simulink model "MIMO_MFDM_Mdl_Zenith"  (R2023b)
settings: Solver=FixedStepAuto  StartTime=0.0  StopTime=tSimStop  FixedStep=0.0004  RelTol=1e-3
values from neighbouring files (symbols this model uses):
  gain_vec_7pts = [g1,g2,g3,g4,g5,g6,g7]'    [mainCompModel_MIMO.m]
  ki = 5    [mainCompModel_MIMO.m]    (also in mainCompModel_SISO.m = 0.3)
  kp = 2000    [mainCompModel_MIMO.m]    (also in mainCompModel_SISO.m = 100)
  m1 = m_tStart(1,1)    [mainCompModel_MIMO.m]
  m2 = m_tStart(2,1)    [mainCompModel_MIMO.m]
  u1 = 0.341009    [mainCompModel_MIMO.m]
  u27 = 0.209818    [mainCompModel_MIMO.m]
undefined symbols (not defined in the file or in its folder): Reference_signals
libraries: cstblocks x4, simulink x4, slpidlib x1
settings Model: Creator=223130458  LastModifiedBy=223130458

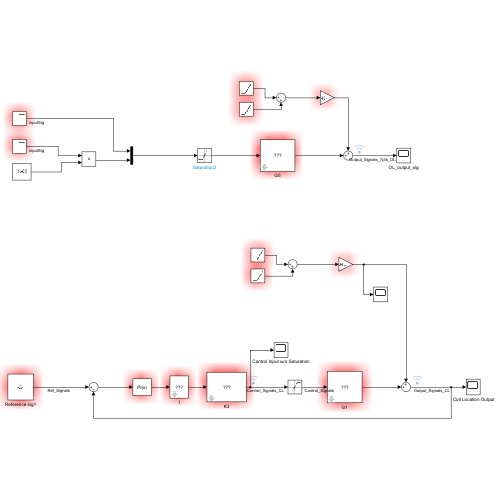
[thumbnail: Simulink's stored preview of the top-level diagram]
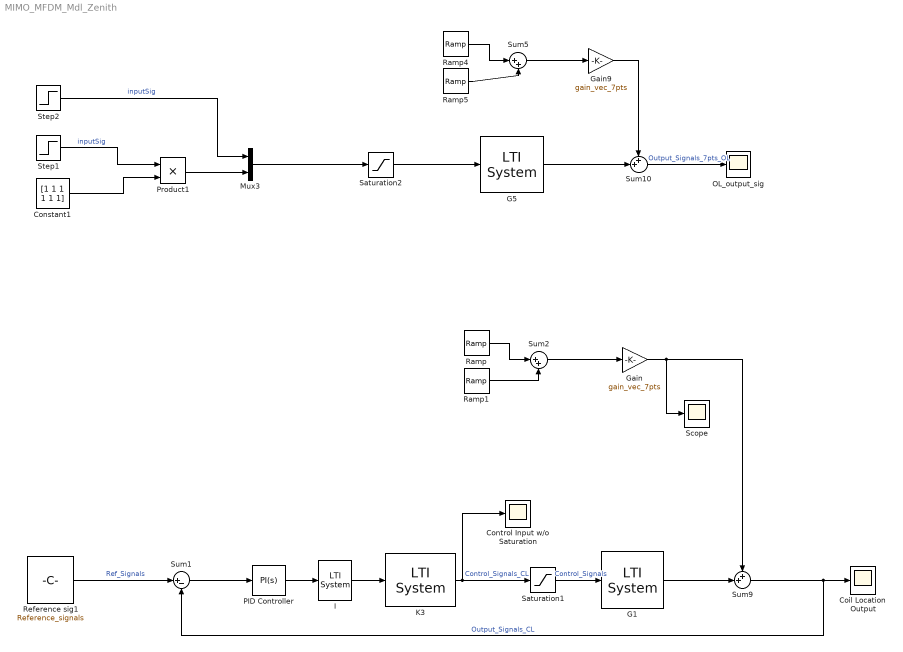
== system MIMO_MFDM_Mdl_Zenith ==
  " Coil Location Output" : Scope
  Constant1 : Constant  Value=[1 1 1 1 1 1]
  Control Input w/o Saturation : Scope
  G1 : cstblocks/LTI System  sys=G  IC=[]  PadeOrder=0
  G5 : cstblocks/LTI System  sys=G  IC=[]  PadeOrder=0
  Gain : Gain  Gain=gain_vec_7pts
  Gain9 : Gain  Gain=gain_vec_7pts
  I : cstblocks/LTI System  sys=I  IC=[]  PadeOrder=0
  K3 : cstblocks/LTI System  sys=G0inv  IC=[]  PadeOrder=0
  Mux3 : Mux  Inputs=2
  OL_output_sig : Scope
  PID Controller : slpidlib/PID Controller  Controller=PI  Form=Parallel  TimeDomain=Continuous-time  UseExternalTs=off  SampleTime=-1  IntegratorMethod=Forward Euler  FilterMethod=Forward Euler  ControllerParametersSource=internal  P=kp  I=ki  UseKiTs=off  D=0  N=100  UseFilter=on  TunerSelectOption=Transfer Function Based (PID Tuner App)  InitialConditionSource=internal  InitialConditionForIntegrator=0  InitialConditionForFilter=0  DifferentiatorICPrevScaledInput=0  ExternalReset=none  TrackingMode=off  Kt=1  LimitOutput=off  SatLimitsSource=internal  UpperSaturationLimit=inf  LowerSaturationLimit=-inf  LinearizeAsGain=on  AntiWindupMode=none  Kb=1  LimitIntegrator=off  UpperIntegratorSaturationLimit=inf  LowerIntegratorSaturationLimit=-inf  POutMin=[]  POutMax=[]  IOutMin=[]  IOutMax=[]  DOutMin=[]  DOutMax=[]  NOutMin=[]  NOutMax=[]  SumOutMin=[]  SumOutMax=[]  SaturationOutMin=[]  SaturationOutMax=[]  PParamMin=[]  PParamMax=[]  IParamMin=[]  IParamMax=[]  DParamMin=[]  DParamMax=[]  NParamMin=[]  NParamMax=[]  KbParamMin=[]  KbParamMax=[]  KtParamMin=[]  KtParamMax=[]  KbOutMin=[]  KbOutMax=[]  KtOutMin=[]  KtOutMax=[]  IntegratorOutMin=[]  IntegratorOutMax=[]  FilterOutMin=[]  FilterOutMax=[]  SumI1OutMin=[]  SumI1OutMax=[]  SumI2OutMin=[]  SumI2OutMax=[]  SumI3OutMin=[]  SumI3OutMax=[]  SumI4OutMin=[]  SumI4OutMax=[]  SumDOutMin=[]  SumDOutMax=[]  DifferentiatorOutMin=[]  DifferentiatorOutMax=[]  FilterDiffOutCoefMin=[]  FilterDiffOutCoefMax=[]  ReciprocalOutMin=[]  ReciprocalOutMax=[]  SumDenOutMin=[]  SumDenOutMax=[]  SumNumOutMin=[]  SumNumOutMax=[]  DivideOutMin=[]  DivideOutMax=[]  UdiffTsProdOutMin=[]  UdiffTsProdOutMax=[]  NTsProdOutMin=[]  NTsProdOutMax=[]  UintegralTsProdOutMin=[]  UintegralTsProdOutMax=[]  UngainTsProdOutMin=[]  UngainTsProdOutMax=[]  ClampingZeroOutDataTypeStr=Inherit: Inherit via back propagation  ClampingZeroOutMin=[]  ClampingZeroOutMax=[]  FilterDenConstantOutDataTypeStr=Inherit: Inherit via back propagation  FilterDenConstantOutMin=[]  FilterDenConstantOutMax=[]  PCopyOutDataTypeStr=Inherit: Inherit via back propagation  PCopyOutMin=[]  PCopyOutMax=[]  NCopyOutDataTypeStr=Inherit: Inherit via back propagation  NCopyOutMin=[]  NCopyOutMax=[]  IntegratorContinuousStateAttributes=''  IntegratorStateMustResolveToSignalObject=off  IntegratorRTWStateStorageClass=Auto  FilterContinuousStateAttributes=''  FilterStateMustResolveToSignalObject=off  FilterRTWStateStorageClass=Auto  ParallelPVariant=InternalParameters  IdealPVariant=Disabled  IVariant=InternalParameters  DVariant=Disabled  IntegratorVariant=Continuous  SatVariant=Disabled  AWVariant=Passthrough  PCopyVariant=Disabled  TRVariant=Disabled  FdbkBlocksVariant=Forward  IdealPFdbkVariant=Disabled  SatFdbkVariant=Disabled  DerivativeFilterVariant=Disabled  NVariant=Disabled  NCopyVariant=Disabled_SignalSpec  FilterICVariant=Disabled  IntegratorICVariant=InternalICs  ExternalResetVariant=Disabled  TRSumVariant=Passthrough  SumFdbkVariant=Disabled  SumVariant=Sum_PI  TsampFilterVariant=InternalTs  TsampNgainVariant=Passthrough  TsampIntegralVariant=Disabled_SignalSpec  ExternalSaturationOutDataTypeStr=Inherit: Same as second input
  Product1 : Product
  Ramp : simulink/Sources/Ramp  slope=m1  start=tStart1  InitialOutput=0
  Ramp1 : simulink/Sources/Ramp  slope=m2  start=tStart2  InitialOutput=0
  Ramp4 : simulink/Sources/Ramp  slope=m1  start=tStart1  InitialOutput=0
  Ramp5 : simulink/Sources/Ramp  slope=m2  start=tStart2  InitialOutput=0
  Reference sig1 : Constant  Value=Reference_signals
  Saturation1 : Saturate  UpperLimit=inf  LowerLimit=-inf
  Saturation2 : Saturate  UpperLimit=inf  LowerLimit=-inf
  Scope : Scope
  Step1 : Step  Time=0  After=u27  SampleTime=0
  Step2 : Step  Time=0  After=u1  SampleTime=0
  Sum1 : Sum  Inputs=|+-
  Sum10 : Sum  Inputs=++|
  Sum2 : Sum  Inputs=|++
  Sum5 : Sum  Inputs=|++
  Sum9 : Sum  Inputs=++|
  wires:
  Sum1/1 -> PID Controller/1
  Reference sig1/1 -> Sum1/1  "Ref_Signals"
  PID Controller/1 -> I/1
  I/1 -> K3/1
  K3/1 -> Saturation1/1, Control Input w/o Saturation/1  "Control_Signals_CL"
  Ramp/1 -> Sum2/1
  Ramp1/1 -> Sum2/2
  G1/1 -> Sum9/2
  Sum9/1 -> Sum1/2, " Coil Location Output"/1  "Output_Signals_CL"
  Product1/1 -> Mux3/2
  Step2/1 -> Mux3/1  "inputSig"
  Constant1/1 -> Product1/2
  Sum10/1 -> OL_output_sig/1  "Output_Signals_7pts_OL"
  Step1/1 -> Product1/1  "inputSig"
  G5/1 -> Sum10/2
  Mux3/1 -> Saturation2/1
  Gain/1 -> Scope/1, Sum9/1
  Saturation1/1 -> G1/1  "Control_Signals"
  Sum2/1 -> Gain/1
  Sum5/1 -> Gain9/1
  Ramp5/1 -> Sum5/2
  Ramp4/1 -> Sum5/1
  Gain9/1 -> Sum10/1
  Saturation2/1 -> G5/1
